simulink model "bounce_ball"  (R2023a)
settings: Solver=ode15s  StartTime=0.0  StopTime=10  MaxStep=.1  RelTol=1e-6  EnableMultiTasking=on
settings Model: Creator=The MathWorks, Inc.  LastModifiedBy=wkmiao
settings SolverCC: ConsecutiveZCsStepRelTol=1*128*eps  ZeroCrossControl=EnableAll  AlgebraicLoopSolver=TrustRegion
settings DataIOCC: SaveFormat=StructureWithTime  ReturnWorkspaceOutputs=off
settings OptimizationCC: ReuseModelBlockBuffer=off  ExpressionDepthLimit=2147483647  InitFltsAndDblsToZero=on  EfficientMapNaN2IntZero=off  LifeSpan=inf
settings DebuggingCC: UnderspecifiedInitializationDetection=Classic  MergeDetectMultiDrivingBlocksExec=none  SignalResolutionControl=TryResolveAllWithWarning  SolverPrmCheckMsg=warning  FcnCallInpInsideContextMsg=warning  UnconnectedInputMsg=warning  UnconnectedOutputMsg=warning  UnconnectedLineMsg=warning  StateNameClashWarn=warning  PregeneratedLibrarySubsystemCodeDiagnostic=none  SFUnexpectedBacktrackingDiag=warning  SFNoUnconditionalDefaultTransitionDiag=warning  SFExecutionAtInitializationDiag=none  ArithmeticOperatorsInVariantConditions=warning
settings HardwareCC: ProdBitPerPointer=32  ProdBitPerSizeT=32  ProdBitPerPtrDiffT=32  ProdLargestAtomicFloat=None  ProdIntDivRoundTo=Undefined  ProdEndianess=Unspecified  ProdWordSize=32  ProdHWDeviceType=32-bit Generic  TargetBitPerPointer=64  TargetBitPerSizeT=64  TargetBitPerPtrDiffT=64  TargetLongLongMode=on  TargetIntDivRoundTo=Zero  TargetEndianess=LittleEndian  TargetWordSize=64  TargetHWDeviceType=MATLAB Host
settings ModelReferenceCC: EnableRefExpFcnMdlSchedulingChecks=on  PropagateSignalLabelsOutOfModel=off
settings SFSimCC: SFSimEcho=off  SimUseLocalCustomCode=off  SimParseCustomCode=off  CustomCodeUndefinedFunction=UseInterfaceOnly
settings RTWCC: RTWUseLocalCustomCode=off  DLArmComputeVersion=19.05
settings CodeAppCC: StateflowObjectComments=on
settings GRTTargetCC: TargetLangStandard=C89/C90 (ANSI)  CombineOutputUpdateFcns=off  GRTInterface=on
settings ConfigComp: CovMetricSettings=dw  CovSaveCumulativeToWorkspaceVar=on  CovSaveSingleToWorkspaceVar=on  CovExternalEMLEnable=off  CovSFcnEnable=off

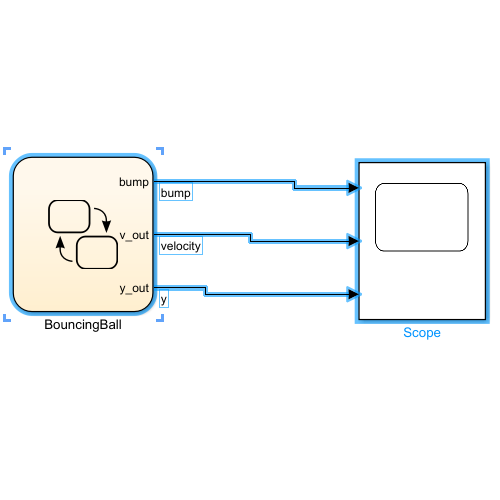
[thumbnail: Simulink's stored preview of the top-level diagram]
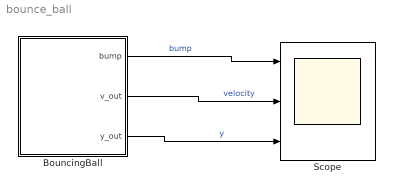
== system bounce_ball ==
  BouncingBall : Stateflow chart  TreatAsAtomicUnit=on
      settings: PortSchema="{\"entries\":[{\"content\":{\"sides\":[{\"content\":{},\"type\":\"ConnectorPlacement.EquallySpacedRectSide\",\"uuid\":\"11c2286e-4f45-42e4-8417-56cd3d10aabd\"},{\"content\":{\"connectorIds\":[\"Out2\",\"Out1\",\"Out3\"],\"side\":\"RIGHT\"},\"type\":\"ConnectorPlacement.EquallySpacedRectSide\",\"uuid\":\"c640f465-3d5f-46ad-9799-96b40f3e223a\"},{\"content\":{\"side\":\"TOP\"},\"type\":\"ConnectorPlacement.EquallySpacedRectSide\",\"uuid\":\"a694eaa9-40a1-47cd-ae9f-ba8686050f54\"}]},\"type\":\"ConnectorPlacement.EquallySpacedConnector\",\"uuid\":\"374e0c11-e06b-4b8c-8e51-1722becc6ff6\"}],\"packageUris\":[\"http://schema.mathworks.com/mf0/Connector/R2020b\"],\"version\":\"1.0\"}"
  Scope : Scope  NumInputPorts=3
  wires:
  BouncingBall/1(v_out) -> Scope/2  "velocity"
  BouncingBall/3(y_out) -> Scope/3  "y"
  BouncingBall/2(bump) -> Scope/1  "bump"

== stateflow chart bounce_ball/BouncingBall ==
  settings: updateMethod=CONTINUOUS  executeAtInitialization=1  initializeOutput=1
  state free
    du:
    % derivatives
    y_dot = v;
    v_dot = -9.81;
    % outputs
    y_out = y;
    v_out = v;
  (default) -> free : {
      | y = 10;
      | v = 0;
      | }
  free -> free : [y <= 0]{
      | bump = 1;
      | y = 0;
      | v = -0.8.*v;
      | }
  data: v_out output double size=1; v local double; bump output double; y local double; y_out output
  data v settings: updateMethod=SF_CONTINUOUS_TIME_DATA
  data y settings: updateMethod=SF_CONTINUOUS_TIME_DATA
